simulink model "NMM_order6_multi3"  (R2023a)
settings: Solver=VariableStepAuto  StartTime=0.0  StopTime=10.0  RelTol=1e-3
undefined symbols (not defined in the file): clf
libraries: simulink x3
(part 2 of 2)

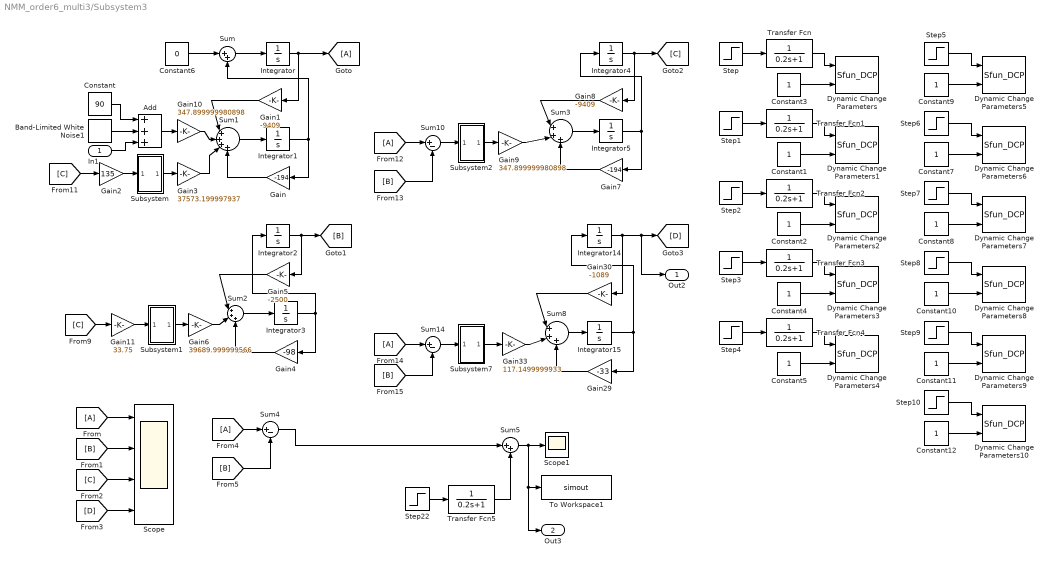
== system NMM_order6_multi3/Subsystem3 ==
  In1 : Inport
  Add : Sum  Inputs=+++
  Band-Limited White Noise1 : simulink/Sources/Band-Limited White Noise  Cov=[0.02]  Ts=0.001  seed=[19361]  VectorParams1D=off
  Constant : Constant  Value=90
  Constant{1..5,7..12} (11 alike) : Constant
  Constant6 : Constant  Value=0
  Dynamic Change Parameters : M-S-Function  StopFcn=close(clf)  FunctionName=Sfun_DCP  Parameters=block_name,par_name,sample_time,dimension  mask{block_name='NMM_order6_multi3/Subsystem3/Gain10', par_name='Gain', reset=off, sample_time=[0.01 0], dimension=[1 1]}
      mask help:
      | Dynamic Change Parameters : Change Block's Parameter When the Model is running
      |
      | block_name : name of the block  need to change parameter,must be string
      | par_name   : name of the parameter want to change,must be string
      | sample_time: sample time of this block
      | demension  : demension of the parameter want to change,must be [m n]
      mask Callback reset:
      | if strcmp( get_param(gcb,'reset'),'on' )
      |    fig_par_set();
      | end
      mask Callback sample_time:
      | st = get_param(gcb,'sample_time');
      | st = str2num(st);
      | if length(st)~=2
      |     msgbox('Sample Time is invalid ');
      | end
      mask Callback dimension:
      | st = get_param(gcb,'dimension');
      | st = str2num(st);
      | if length(st)~=2
      |     msgbox('Fromat of Dimension must be [m n]');
      | end
  Dynamic Change Parameters1 : M-S-Function  StopFcn=close(clf)  FunctionName=Sfun_DCP  Parameters=block_name,par_name,sample_time,dimension  mask{block_name='NMM_order6_multi3/Subsystem3/Gain3', par_name='Gain', reset=off, sample_time=[0.01 0], dimension=[1 1]}
      mask help:
      | Dynamic Change Parameters : Change Block's Parameter When the Model is running
      |
      | block_name : name of the block  need to change parameter,must be string
      | par_name   : name of the parameter want to change,must be string
      | sample_time: sample time of this block
      | demension  : demension of the parameter want to change,must be [m n]
      mask Callback reset:
      | if strcmp( get_param(gcb,'reset'),'on' )
      |    fig_par_set();
      | end
      mask Callback sample_time:
      | st = get_param(gcb,'sample_time');
      | st = str2num(st);
      | if length(st)~=2
      |     msgbox('Sample Time is invalid ');
      | end
      mask Callback dimension:
      | st = get_param(gcb,'dimension');
      | st = str2num(st);
      | if length(st)~=2
      |     msgbox('Fromat of Dimension must be [m n]');
      | end
  Dynamic Change Parameters10 : M-S-Function  StopFcn=close(clf)  FunctionName=Sfun_DCP  Parameters=block_name,par_name,sample_time,dimension  mask{block_name='NMM_order6_multi3/Subsystem3/Gain7', par_name='Gain', reset=off, sample_time=[0.01 0], dimension=[1 1]}
      mask help:
      | Dynamic Change Parameters : Change Block's Parameter When the Model is running
      |
      | block_name : name of the block  need to change parameter,must be string
      | par_name   : name of the parameter want to change,must be string
      | sample_time: sample time of this block
      | demension  : demension of the parameter want to change,must be [m n]
      mask Callback reset:
      | if strcmp( get_param(gcb,'reset'),'on' )
      |    fig_par_set();
      | end
      mask Callback sample_time:
      | st = get_param(gcb,'sample_time');
      | st = str2num(st);
      | if length(st)~=2
      |     msgbox('Sample Time is invalid ');
      | end
      mask Callback dimension:
      | st = get_param(gcb,'dimension');
      | st = str2num(st);
      | if length(st)~=2
      |     msgbox('Fromat of Dimension must be [m n]');
      | end
  Dynamic Change Parameters2 : M-S-Function  StopFcn=close(clf)  FunctionName=Sfun_DCP  Parameters=block_name,par_name,sample_time,dimension  mask{block_name='NMM_order6_multi3/Subsystem3/Gain6', par_name='Gain', reset=off, sample_time=[0.01 0], dimension=[1 1]}
      mask help:
      | Dynamic Change Parameters : Change Block's Parameter When the Model is running
      |
      | block_name : name of the block  need to change parameter,must be string
      | par_name   : name of the parameter want to change,must be string
      | sample_time: sample time of this block
      | demension  : demension of the parameter want to change,must be [m n]
      mask Callback reset:
      | if strcmp( get_param(gcb,'reset'),'on' )
      |    fig_par_set();
      | end
      mask Callback sample_time:
      | st = get_param(gcb,'sample_time');
      | st = str2num(st);
      | if length(st)~=2
      |     msgbox('Sample Time is invalid ');
      | end
      mask Callback dimension:
      | st = get_param(gcb,'dimension');
      | st = str2num(st);
      | if length(st)~=2
      |     msgbox('Fromat of Dimension must be [m n]');
      | end
  Dynamic Change Parameters3 : M-S-Function  StopFcn=close(clf)  FunctionName=Sfun_DCP  Parameters=block_name,par_name,sample_time,dimension  mask{block_name='NMM_order6_multi3/Subsystem3/Gain9', par_name='Gain', reset=off, sample_time=[0.01 0], dimension=[1 1]}
      mask help:
      | Dynamic Change Parameters : Change Block's Parameter When the Model is running
      |
      | block_name : name of the block  need to change parameter,must be string
      | par_name   : name of the parameter want to change,must be string
      | sample_time: sample time of this block
      | demension  : demension of the parameter want to change,must be [m n]
      mask Callback reset:
      | if strcmp( get_param(gcb,'reset'),'on' )
      |    fig_par_set();
      | end
      mask Callback sample_time:
      | st = get_param(gcb,'sample_time');
      | st = str2num(st);
      | if length(st)~=2
      |     msgbox('Sample Time is invalid ');
      | end
      mask Callback dimension:
      | st = get_param(gcb,'dimension');
      | st = str2num(st);
      | if length(st)~=2
      |     msgbox('Fromat of Dimension must be [m n]');
      | end
  Dynamic Change Parameters4 : M-S-Function  StopFcn=close(clf)  FunctionName=Sfun_DCP  Parameters=block_name,par_name,sample_time,dimension  mask{block_name='NMM_order6_multi3/Subsystem3/Gain33', par_name='Gain', reset=off, sample_time=[0.01 0], dimension=[1 1]}
      mask help:
      | Dynamic Change Parameters : Change Block's Parameter When the Model is running
      |
      | block_name : name of the block  need to change parameter,must be string
      | par_name   : name of the parameter want to change,must be string
      | sample_time: sample time of this block
      | demension  : demension of the parameter want to change,must be [m n]
      mask Callback reset:
      | if strcmp( get_param(gcb,'reset'),'on' )
      |    fig_par_set();
      | end
      mask Callback sample_time:
      | st = get_param(gcb,'sample_time');
      | st = str2num(st);
      | if length(st)~=2
      |     msgbox('Sample Time is invalid ');
      | end
      mask Callback dimension:
      | st = get_param(gcb,'dimension');
      | st = str2num(st);
      | if length(st)~=2
      |     msgbox('Fromat of Dimension must be [m n]');
      | end
  Dynamic Change Parameters5 : M-S-Function  StopFcn=close(clf)  FunctionName=Sfun_DCP  Parameters=block_name,par_name,sample_time,dimension  mask{block_name='NMM_order6_multi3/Subsystem3/Gain1', par_name='Gain', reset=off, sample_time=[0.01 0], dimension=[1 1]}
      mask help:
      | Dynamic Change Parameters : Change Block's Parameter When the Model is running
      |
      | block_name : name of the block  need to change parameter,must be string
      | par_name   : name of the parameter want to change,must be string
      | sample_time: sample time of this block
      | demension  : demension of the parameter want to change,must be [m n]
      mask Callback reset:
      | if strcmp( get_param(gcb,'reset'),'on' )
      |    fig_par_set();
      | end
      mask Callback sample_time:
      | st = get_param(gcb,'sample_time');
      | st = str2num(st);
      | if length(st)~=2
      |     msgbox('Sample Time is invalid ');
      | end
      mask Callback dimension:
      | st = get_param(gcb,'dimension');
      | st = str2num(st);
      | if length(st)~=2
      |     msgbox('Fromat of Dimension must be [m n]');
      | end
  Dynamic Change Parameters6 : M-S-Function  StopFcn=close(clf)  FunctionName=Sfun_DCP  Parameters=block_name,par_name,sample_time,dimension  mask{block_name='NMM_order6_multi3/Subsystem3/Gain', par_name='Gain', reset=off, sample_time=[0.01 0], dimension=[1 1]}
      mask help:
      | Dynamic Change Parameters : Change Block's Parameter When the Model is running
      |
      | block_name : name of the block  need to change parameter,must be string
      | par_name   : name of the parameter want to change,must be string
      | sample_time: sample time of this block
      | demension  : demension of the parameter want to change,must be [m n]
      mask Callback reset:
      | if strcmp( get_param(gcb,'reset'),'on' )
      |    fig_par_set();
      | end
      mask Callback sample_time:
      | st = get_param(gcb,'sample_time');
      | st = str2num(st);
      | if length(st)~=2
      |     msgbox('Sample Time is invalid ');
      | end
      mask Callback dimension:
      | st = get_param(gcb,'dimension');
      | st = str2num(st);
      | if length(st)~=2
      |     msgbox('Fromat of Dimension must be [m n]');
      | end
  Dynamic Change Parameters7 : M-S-Function  StopFcn=close(clf)  FunctionName=Sfun_DCP  Parameters=block_name,par_name,sample_time,dimension  mask{block_name='NMM_order6_multi3/Subsystem3/Gain5', par_name='Gain', reset=off, sample_time=[0.01 0], dimension=[1 1]}
      mask help:
      | Dynamic Change Parameters : Change Block's Parameter When the Model is running
      |
      | block_name : name of the block  need to change parameter,must be string
      | par_name   : name of the parameter want to change,must be string
      | sample_time: sample time of this block
      | demension  : demension of the parameter want to change,must be [m n]
      mask Callback reset:
      | if strcmp( get_param(gcb,'reset'),'on' )
      |    fig_par_set();
      | end
      mask Callback sample_time:
      | st = get_param(gcb,'sample_time');
      | st = str2num(st);
      | if length(st)~=2
      |     msgbox('Sample Time is invalid ');
      | end
      mask Callback dimension:
      | st = get_param(gcb,'dimension');
      | st = str2num(st);
      | if length(st)~=2
      |     msgbox('Fromat of Dimension must be [m n]');
      | end
  Dynamic Change Parameters8 : M-S-Function  StopFcn=close(clf)  FunctionName=Sfun_DCP  Parameters=block_name,par_name,sample_time,dimension  mask{block_name='NMM_order6_multi3/Subsystem3/Gain4', par_name='Gain', reset=off, sample_time=[0.01 0], dimension=[1 1]}
      mask help:
      | Dynamic Change Parameters : Change Block's Parameter When the Model is running
      |
      | block_name : name of the block  need to change parameter,must be string
      | par_name   : name of the parameter want to change,must be string
      | sample_time: sample time of this block
      | demension  : demension of the parameter want to change,must be [m n]
      mask Callback reset:
      | if strcmp( get_param(gcb,'reset'),'on' )
      |    fig_par_set();
      | end
      mask Callback sample_time:
      | st = get_param(gcb,'sample_time');
      | st = str2num(st);
      | if length(st)~=2
      |     msgbox('Sample Time is invalid ');
      | end
      mask Callback dimension:
      | st = get_param(gcb,'dimension');
      | st = str2num(st);
      | if length(st)~=2
      |     msgbox('Fromat of Dimension must be [m n]');
      | end
  Dynamic Change Parameters9 : M-S-Function  StopFcn=close(clf)  FunctionName=Sfun_DCP  Parameters=block_name,par_name,sample_time,dimension  mask{block_name='NMM_order6_multi3/Subsystem3/Gain8', par_name='Gain', reset=off, sample_time=[0.01 0], dimension=[1 1]}
      mask help:
      | Dynamic Change Parameters : Change Block's Parameter When the Model is running
      |
      | block_name : name of the block  need to change parameter,must be string
      | par_name   : name of the parameter want to change,must be string
      | sample_time: sample time of this block
      | demension  : demension of the parameter want to change,must be [m n]
      mask Callback reset:
      | if strcmp( get_param(gcb,'reset'),'on' )
      |    fig_par_set();
      | end
      mask Callback sample_time:
      | st = get_param(gcb,'sample_time');
      | st = str2num(st);
      | if length(st)~=2
      |     msgbox('Sample Time is invalid ');
      | end
      mask Callback dimension:
      | st = get_param(gcb,'dimension');
      | st = str2num(st);
      | if length(st)~=2
      |     msgbox('Fromat of Dimension must be [m n]');
      | end
  From{,4,12,14} (4 alike) : From
  Gain : Gain  Gain=-194
  Gain1 : Gain  Gain=-9409
  Gain10 : Gain  Gain=347.899999980898
  Gain11 : Gain  Gain=33.75
  Gain2 : Gain  Gain=135
  Gain29 : Gain  Gain=-33
  Gain3 : Gain  Gain=37573.199997937
  Gain30 : Gain  Gain=-1089
  Gain33 : Gain  Gain=117.1499999933
  Gain4 : Gain  Gain=-98
  Gain5 : Gain  Gain=-2500
  Gain6 : Gain  Gain=39689.999999566
  Gain7 : Gain  Gain=-194
  Gain8 : Gain  Gain=-9409
  Gain9 : Gain  Gain=347.899999980898
  Goto : Goto
  Integrator{,1..5,14..15} (8 alike) : Integrator
  Scope : Scope  NumInputPorts=4
  Scope1 : Scope
  Step : Step  Time=5.5  Before=2.35*100  After=3.55*98  SampleTime=0
  Step1 : Step  Time=5.5  Before=2.35*100*108  After=3.55*98*108  SampleTime=0
  Step10 : Step  Time=5.5  Before=-200  After=-194  SampleTime=0
  Step2 : Step  Time=5.5  Before=22*50*33.75  After=24*49*33.75  SampleTime=0
  Step22 : Step  Time=6.0  After=0.2  SampleTime=0
  Step3 : Step  Time=5.5  Before=2.35*100  After=3.55*98  SampleTime=0
  Step4 : Step  Time=5.5  Before=2.35*33  After=3.55*33  SampleTime=0
  Step5 : Step  Time=5.5  Before=-10000  After=-9409  SampleTime=0
  Step6 : Step  Time=5.5  Before=-200  After=-194  SampleTime=0
  Step7 : Step  Time=100  Before=-2500  After=-2451  SampleTime=0
  Step8 : Step  Time=5.5  Before=-100  After=-98  SampleTime=0
  Step9 : Step  Time=5.5  Before=-10000  After=-9409  SampleTime=0
  Subsystem : Subsystem
  Subsystem1 : Subsystem
  Subsystem2 : Subsystem
  Subsystem7 : Subsystem
  Sum : Sum  Inputs=|++
  Sum1 : Sum  Inputs=|++++
  Sum10 : Sum  Inputs=|+-
  Sum14 : Sum  Inputs=|+-
  Sum2 : Sum  Inputs=|+++
  Sum3 : Sum  Inputs=|+++
  Sum4 : Sum  Inputs=|+-
  Sum5 : Sum  Inputs=|++
  Sum8 : Sum  Inputs=|+++
  To Workspace1 : ToWorkspace  VariableName=simout  SaveFormat=Timeseries  SampleTime=-1
  Transfer Fcn{,1..5} (6 alike) : TransferFcn  Denominator=[0.2 1]
  Out2 : Outport
  Out3 : Outport  Port=2
  wires:
  From4/1 -> Sum4/1
  Integrator5/1 -> Gain7/1, Integrator4/1
  Integrator1/1 -> Sum/2, Gain/1
  [B] -> Sum4/2
  Gain33/1 -> Sum8/2
  Gain30/1 -> Sum8/1
  Integrator15/1 -> Gain29/1, Integrator14/1
  [B] -> Scope/2
  Gain11/1 -> Subsystem1/1(In1)
  Integrator/1 -> Goto/1, Gain1/1
  From12/1 -> Sum10/1
  Subsystem/1(Out2) -> Gain3/1
  Sum8/1 -> Integrator15/1
  Gain1/1 -> Sum1/1
  [B] -> Sum14/2
  Gain4/1 -> Sum2/3
  From/1 -> Scope/1
  [C] -> Gain11/1
  Sum3/1 -> Integrator5/1
  Gain8/1 -> Sum3/1
  Subsystem7/1(Out2) -> Gain33/1
  Sum4/1 -> Sum5/1
  Integrator3/1 -> Gain4/1, Integrator2/1
  Constant/1 -> Add/1
  Gain2/1 -> Subsystem/1(In1)
  Gain7/1 -> Sum3/3
  Gain10/1 -> Sum1/2
  [C] -> Scope/3
  Subsystem2/1(Out2) -> Gain9/1
  Integrator14/1 -> [D], Out2/1, Gain30/1
  Subsystem1/1(Out2) -> Gain6/1
  Sum2/1 -> Integrator3/1
  Add/1 -> Gain10/1
  Sum10/1 -> Subsystem2/1(In1)
  From14/1 -> Sum14/1
  Sum1/1 -> Integrator1/1
  Sum/1 -> Integrator/1
  [D] -> Scope/4
  Integrator4/1 -> [C], Gain8/1
  Gain3/1 -> Sum1/3
  [B] -> Sum10/2
  Gain9/1 -> Sum3/2
  Gain6/1 -> Sum2/2
  Sum14/1 -> Subsystem7/1(In1)
  [C] -> Gain2/1
  Gain29/1 -> Sum8/3
  Band-Limited White Noise1/1 -> Add/2
  Constant6/1 -> Sum/1
  Gain5/1 -> Sum2/1
  Integrator2/1 -> [B], Gain5/1
  Gain/1 -> Sum1/4
  In1/1 -> Add/3
  Constant4/1 -> Dynamic Change Parameters3/2
  Constant1/1 -> Dynamic Change Parameters1/2
  Constant3/1 -> Dynamic Change Parameters/2
  Constant5/1 -> Dynamic Change Parameters4/2
  Constant2/1 -> Dynamic Change Parameters2/2
  Step/1 -> Transfer Fcn/1
  Transfer Fcn/1 -> Dynamic Change Parameters/1
  Transfer Fcn1/1 -> Dynamic Change Parameters1/1
  Step1/1 -> Transfer Fcn1/1
  Transfer Fcn2/1 -> Dynamic Change Parameters2/1
  Step2/1 -> Transfer Fcn2/1
  Transfer Fcn3/1 -> Dynamic Change Parameters3/1
  Step3/1 -> Transfer Fcn3/1
  Transfer Fcn4/1 -> Dynamic Change Parameters4/1
  Step4/1 -> Transfer Fcn4/1
  Constant7/1 -> Dynamic Change Parameters6/2
  Constant10/1 -> Dynamic Change Parameters8/2
  Step9/1 -> Dynamic Change Parameters9/1
  Step5/1 -> Dynamic Change Parameters5/1
  Step8/1 -> Dynamic Change Parameters8/1
  Constant8/1 -> Dynamic Change Parameters7/2
  Constant11/1 -> Dynamic Change Parameters9/2
  Step7/1 -> Dynamic Change Parameters7/1
  Step6/1 -> Dynamic Change Parameters6/1
  Constant9/1 -> Dynamic Change Parameters5/2
  Step10/1 -> Dynamic Change Parameters10/1
  Constant12/1 -> Dynamic Change Parameters10/2
  Sum5/1 -> Scope1/1, Out3/1, To Workspace1/1
  Step22/1 -> Transfer Fcn5/1
  Transfer Fcn5/1 -> Sum5/2

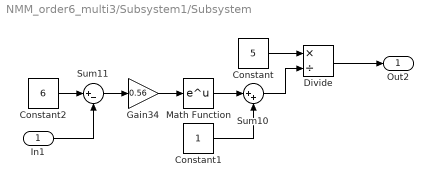
== system NMM_order6_multi3/Subsystem1/Subsystem ==
  In1 : Inport
  Constant : Constant  Value=5
  Constant1 : Constant
  Constant2 : Constant  Value=6
  Divide : Product  Inputs=*/
  Gain34 : Gain  Gain=0.56
  Math Function : Math
  Sum10 : Sum  Inputs=|++
  Sum11 : Sum  Inputs=|+-
  Out2 : Outport
  wires:
  Sum11/1 -> Gain34/1
  Constant/1 -> Divide/1
  Math Function/1 -> Sum10/1
  Constant2/1 -> Sum11/1
  In1/1 -> Sum11/2
  Divide/1 -> Out2/1
  Gain34/1 -> Math Function/1
  Constant1/1 -> Sum10/2
  Sum10/1 -> Divide/2

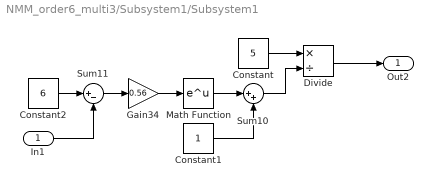
== system NMM_order6_multi3/Subsystem1/Subsystem1 ==
  In1 : Inport
  Constant : Constant  Value=5
  Constant1 : Constant
  Constant2 : Constant  Value=6
  Divide : Product  Inputs=*/
  Gain34 : Gain  Gain=0.56
  Math Function : Math
  Sum10 : Sum  Inputs=|++
  Sum11 : Sum  Inputs=|+-
  Out2 : Outport
  wires:
  Sum11/1 -> Gain34/1
  Constant/1 -> Divide/1
  Math Function/1 -> Sum10/1
  Constant2/1 -> Sum11/1
  In1/1 -> Sum11/2
  Divide/1 -> Out2/1
  Gain34/1 -> Math Function/1
  Constant1/1 -> Sum10/2
  Sum10/1 -> Divide/2

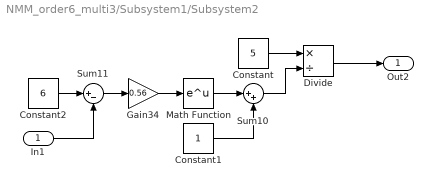
== system NMM_order6_multi3/Subsystem1/Subsystem2 ==
  In1 : Inport
  Constant : Constant  Value=5
  Constant1 : Constant
  Constant2 : Constant  Value=6
  Divide : Product  Inputs=*/
  Gain34 : Gain  Gain=0.56
  Math Function : Math
  Sum10 : Sum  Inputs=|++
  Sum11 : Sum  Inputs=|+-
  Out2 : Outport
  wires:
  Sum11/1 -> Gain34/1
  Constant/1 -> Divide/1
  Math Function/1 -> Sum10/1
  Constant2/1 -> Sum11/1
  In1/1 -> Sum11/2
  Divide/1 -> Out2/1
  Gain34/1 -> Math Function/1
  Constant1/1 -> Sum10/2
  Sum10/1 -> Divide/2

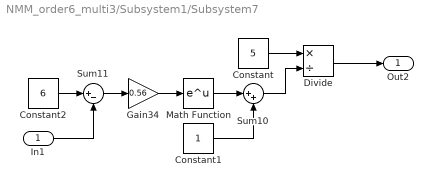
== system NMM_order6_multi3/Subsystem1/Subsystem7 ==
  In1 : Inport
  Constant : Constant  Value=5
  Constant1 : Constant
  Constant2 : Constant  Value=6
  Divide : Product  Inputs=*/
  Gain34 : Gain  Gain=0.56
  Math Function : Math
  Sum10 : Sum  Inputs=|++
  Sum11 : Sum  Inputs=|+-
  Out2 : Outport
  wires:
  Sum11/1 -> Gain34/1
  Constant/1 -> Divide/1
  Math Function/1 -> Sum10/1
  Constant2/1 -> Sum11/1
  In1/1 -> Sum11/2
  Divide/1 -> Out2/1
  Gain34/1 -> Math Function/1
  Constant1/1 -> Sum10/2
  Sum10/1 -> Divide/2

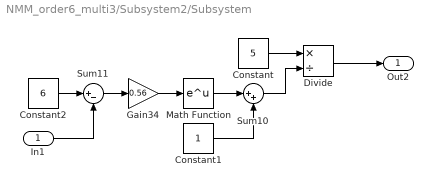
== system NMM_order6_multi3/Subsystem2/Subsystem ==
  In1 : Inport
  Constant : Constant  Value=5
  Constant1 : Constant
  Constant2 : Constant  Value=6
  Divide : Product  Inputs=*/
  Gain34 : Gain  Gain=0.56
  Math Function : Math
  Sum10 : Sum  Inputs=|++
  Sum11 : Sum  Inputs=|+-
  Out2 : Outport
  wires:
  Sum11/1 -> Gain34/1
  Constant/1 -> Divide/1
  Math Function/1 -> Sum10/1
  Constant2/1 -> Sum11/1
  In1/1 -> Sum11/2
  Divide/1 -> Out2/1
  Gain34/1 -> Math Function/1
  Constant1/1 -> Sum10/2
  Sum10/1 -> Divide/2

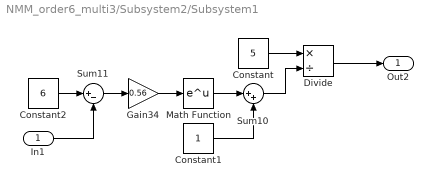
== system NMM_order6_multi3/Subsystem2/Subsystem1 ==
  In1 : Inport
  Constant : Constant  Value=5
  Constant1 : Constant
  Constant2 : Constant  Value=6
  Divide : Product  Inputs=*/
  Gain34 : Gain  Gain=0.56
  Math Function : Math
  Sum10 : Sum  Inputs=|++
  Sum11 : Sum  Inputs=|+-
  Out2 : Outport
  wires:
  Sum11/1 -> Gain34/1
  Constant/1 -> Divide/1
  Math Function/1 -> Sum10/1
  Constant2/1 -> Sum11/1
  In1/1 -> Sum11/2
  Divide/1 -> Out2/1
  Gain34/1 -> Math Function/1
  Constant1/1 -> Sum10/2
  Sum10/1 -> Divide/2

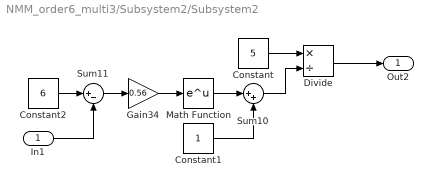
== system NMM_order6_multi3/Subsystem2/Subsystem2 ==
  In1 : Inport
  Constant : Constant  Value=5
  Constant1 : Constant
  Constant2 : Constant  Value=6
  Divide : Product  Inputs=*/
  Gain34 : Gain  Gain=0.56
  Math Function : Math
  Sum10 : Sum  Inputs=|++
  Sum11 : Sum  Inputs=|+-
  Out2 : Outport
  wires:
  Sum11/1 -> Gain34/1
  Constant/1 -> Divide/1
  Math Function/1 -> Sum10/1
  Constant2/1 -> Sum11/1
  In1/1 -> Sum11/2
  Divide/1 -> Out2/1
  Gain34/1 -> Math Function/1
  Constant1/1 -> Sum10/2
  Sum10/1 -> Divide/2

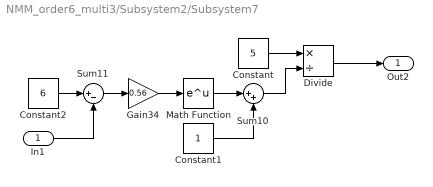
== system NMM_order6_multi3/Subsystem2/Subsystem7 ==
  In1 : Inport
  Constant : Constant  Value=5
  Constant1 : Constant
  Constant2 : Constant  Value=6
  Divide : Product  Inputs=*/
  Gain34 : Gain  Gain=0.56
  Math Function : Math
  Sum10 : Sum  Inputs=|++
  Sum11 : Sum  Inputs=|+-
  Out2 : Outport
  wires:
  Sum11/1 -> Gain34/1
  Constant/1 -> Divide/1
  Math Function/1 -> Sum10/1
  Constant2/1 -> Sum11/1
  In1/1 -> Sum11/2
  Divide/1 -> Out2/1
  Gain34/1 -> Math Function/1
  Constant1/1 -> Sum10/2
  Sum10/1 -> Divide/2

== system NMM_order6_multi3/Subsystem3/Subsystem ==
  In1 : Inport
  Constant : Constant  Value=5
  Constant1 : Constant
  Constant2 : Constant  Value=6
  Divide : Product  Inputs=*/
  Gain34 : Gain  Gain=0.56
  Math Function : Math
  Sum10 : Sum  Inputs=|++
  Sum11 : Sum  Inputs=|+-
  Out2 : Outport
  wires:
  Sum11/1 -> Gain34/1
  Constant/1 -> Divide/1
  Math Function/1 -> Sum10/1
  Constant2/1 -> Sum11/1
  In1/1 -> Sum11/2
  Divide/1 -> Out2/1
  Gain34/1 -> Math Function/1
  Constant1/1 -> Sum10/2
  Sum10/1 -> Divide/2

== system NMM_order6_multi3/Subsystem3/Subsystem1 ==
  In1 : Inport
  Constant : Constant  Value=5
  Constant1 : Constant
  Constant2 : Constant  Value=6
  Divide : Product  Inputs=*/
  Gain34 : Gain  Gain=0.56
  Math Function : Math
  Sum10 : Sum  Inputs=|++
  Sum11 : Sum  Inputs=|+-
  Out2 : Outport
  wires:
  Sum11/1 -> Gain34/1
  Constant/1 -> Divide/1
  Math Function/1 -> Sum10/1
  Constant2/1 -> Sum11/1
  In1/1 -> Sum11/2
  Divide/1 -> Out2/1
  Gain34/1 -> Math Function/1
  Constant1/1 -> Sum10/2
  Sum10/1 -> Divide/2

== system NMM_order6_multi3/Subsystem3/Subsystem2 ==
  In1 : Inport
  Constant : Constant  Value=5
  Constant1 : Constant
  Constant2 : Constant  Value=6
  Divide : Product  Inputs=*/
  Gain34 : Gain  Gain=0.56
  Math Function : Math
  Sum10 : Sum  Inputs=|++
  Sum11 : Sum  Inputs=|+-
  Out2 : Outport
  wires:
  Sum11/1 -> Gain34/1
  Constant/1 -> Divide/1
  Math Function/1 -> Sum10/1
  Constant2/1 -> Sum11/1
  In1/1 -> Sum11/2
  Divide/1 -> Out2/1
  Gain34/1 -> Math Function/1
  Constant1/1 -> Sum10/2
  Sum10/1 -> Divide/2

== system NMM_order6_multi3/Subsystem3/Subsystem7 ==
  In1 : Inport
  Constant : Constant  Value=5
  Constant1 : Constant
  Constant2 : Constant  Value=6
  Divide : Product  Inputs=*/
  Gain34 : Gain  Gain=0.56
  Math Function : Math
  Sum10 : Sum  Inputs=|++
  Sum11 : Sum  Inputs=|+-
  Out2 : Outport
  wires:
  Sum11/1 -> Gain34/1
  Constant/1 -> Divide/1
  Math Function/1 -> Sum10/1
  Constant2/1 -> Sum11/1
  In1/1 -> Sum11/2
  Divide/1 -> Out2/1
  Gain34/1 -> Math Function/1
  Constant1/1 -> Sum10/2
  Sum10/1 -> Divide/2
